simulink model "UZ_EnDat_be4_optimizing_agaib"  (R2023b)
settings: Solver=FixedStepDiscrete  StartTime=0  StopTime=0.002  RelTol=1e-3
model workspace (MAT data in the model file):
  Select = 0
libraries: hdlsllib x750, simulink x19, simulink_extras x4
(part 3 of 9)

== system UZ_EnDat_be4_optimizing_agaib/UZ_ENDAT/responseslicer5 ==
  DATA : Inport  OutDataTypeStr=uint64
  Bit Slice : hdlsllib/Logic and Bit Operations/Bit Slice  Commented=on  lidx=15  ridx=0
  Bit Slice1 : hdlsllib/Logic and Bit Operations/Bit Slice  Commented=on  lidx=63  ridx=48
  Bit Slice2 : hdlsllib/Logic and Bit Operations/Bit Slice  Commented=on  lidx=47  ridx=44
  Bit Slice3 : hdlsllib/Logic and Bit Operations/Bit Slice  lidx=43  ridx=39
  Bit Slice4 : hdlsllib/Logic and Bit Operations/Bit Slice  lidx=38  ridx=16
  Data Type Conversion : DataTypeConversion  Commented=on  OutDataTypeStr=uint16  SaturateOnIntegerOverflow=off  RndMeth=Floor
  Data Type Conversion1 : DataTypeConversion  Commented=on  OutDataTypeStr=uint16  SaturateOnIntegerOverflow=off  RndMeth=Floor
  Data Type Conversion2 : DataTypeConversion  Commented=through  OutDataTypeStr=uint8  SaturateOnIntegerOverflow=off  RndMeth=Floor
  Data Type Conversion3 : DataTypeConversion  OutDataTypeStr=uint8  SaturateOnIntegerOverflow=off  RndMeth=Floor
  Data Type Conversion4 : DataTypeConversion  OutDataTypeStr=uint32  SaturateOnIntegerOverflow=off  RndMeth=Floor
  ENDAT23BITREVERSER : Subsystem  Commented=on
  upppadding : Outport  OutDataTypeStr=uint16
  lowpadding : Outport  Port=2  OutDataTypeStr=uint16
  upperrecivervalue : Outport  Port=3  OutDataTypeStr=uint8
  CRC : Outport  Port=4  OutDataTypeStr=uint8
  payload : Outport  Port=5  OutDataTypeStr=uint32
  wires:
  DATA/1 -> Bit Slice4/1, Bit Slice3/1
  Bit Slice/1 -> Data Type Conversion/1
  Bit Slice1/1 -> Data Type Conversion1/1
  Data Type Conversion/1 -> lowpadding/1
  Data Type Conversion1/1 -> upppadding/1
  Bit Slice3/1 -> Data Type Conversion3/1
  Bit Slice2/1 -> Data Type Conversion2/1
  Bit Slice4/1 -> ENDAT23BITREVERSER/1(in), Data Type Conversion4/1
  Data Type Conversion2/1 -> upperrecivervalue/1
  Data Type Conversion3/1 -> CRC/1
  Data Type Conversion4/1 -> payload/1

== system UZ_EnDat_be4_optimizing_agaib/UZ_ENDAT/timingprovider ==
  wrok : Inport  OutDataTypeStr=boolean
  clk : Inport  Port=2  OutDataTypeStr=boolean
  CLKCNTER_POSCNTR : Subsystem
      settings: LibrarySourceBlock=|
      | hdlsllib/Ports &
      | Subsystems/Subsystem
  CLKCNTER_POSCNTR1 : Subsystem
      settings: LibrarySourceBlock=|
      | hdlsllib/Ports &
      | Subsystems/Subsystem
  Compare To Constant : hdlsllib/Logic and Bit Operations/Compare To Constant  relop=>  const=3  OutDataTypeStr=boolean
  Compare To Constant1 : hdlsllib/Logic and Bit Operations/Compare To Constant  relop===  const=0  OutDataTypeStr=boolean
  Constant3 : Constant  Commented=on  Value=0x7FFFF0  OutDataTypeStr=uint32  SampleTime=-1
  Constant4 : Constant  Commented=on  Value=0x7FFFFF  OutDataTypeStr=uint32  SampleTime=-1
  Detect Increase1 : simulink/Logic and Bit Operations/Detect Increase  vinit=0.0  OutDataTypeStr=boolean
      settings: LibrarySourceBlock=|
      | hdlsllib/Logic and Bit
      | Operations/Detect
      | Increase
  Logical Operator : Logic  Operator=OR  AllPortsSameDT=off  OutDataTypeStr=boolean
  Scope : Scope  NumInputPorts=2
  Subsystem2 : Subsystem
  Subsystem3 : Subsystem
  Subsystem4 : Subsystem  Commented=on
  timeelapsed2cycl : Outport  OutDataTypeStr=uint32
  timeelapsed1cycl : Outport  Port=2  OutDataTypeStr=uint32
  wires:
  clk/1 -> CLKCNTER_POSCNTR1/1(CLK), Subsystem4/1(countclk), CLKCNTER_POSCNTR/2(CLK2CNT), CLKCNTER_POSCNTR/1(CLK)
  wrok/1 -> Detect Increase1/1
  Detect Increase1/1 -> CLKCNTER_POSCNTR1/2(CLK2CNT)
  CLKCNTER_POSCNTR/1(CNT) -> Scope/1, Subsystem3/2(clkcnt), Subsystem2/2(clkcnt)
  Subsystem2/1(ns elapsed) -> timeelapsed2cycl/1
  Subsystem3/1(ns elapsed) -> Scope/2, timeelapsed1cycl/1
  CLKCNTER_POSCNTR1/1(CNT) -> Subsystem3/1(elapsed), Subsystem2/1(elapsed), Compare To Constant/1, Compare To Constant1/1
  Compare To Constant/1 -> Logical Operator/1, CLKCNTER_POSCNTR1/3(ResetCNT)
  Logical Operator/1 -> Subsystem4/2(reset), CLKCNTER_POSCNTR/3(ResetCNT)
  Compare To Constant1/1 -> Logical Operator/2

== system UZ_EnDat_be4_optimizing_agaib/UZ_ENDAT/3timestorage/Storage1 ==
  Data : Inport
  Write : Inport  Port=2  OutDataTypeStr=boolean
  Delay2 : Delay  DelayLength=1
  Switch : Switch  Criteria=u2 > Threshold  SaturateOnIntegerOverflow=off  InputSameDT=off
  out : Outport
  wires:
  Switch/1 -> Delay2/1, out/1
  Delay2/1 -> Switch/3
  Data/1 -> Switch/1
  Write/1 -> Switch/2

== system UZ_EnDat_be4_optimizing_agaib/UZ_ENDAT/3timestorage/Storage2 ==
  Data : Inport
  Write : Inport  Port=2  OutDataTypeStr=boolean
  Delay2 : Delay  DelayLength=1
  Switch : Switch  Criteria=u2 > Threshold  SaturateOnIntegerOverflow=off  InputSameDT=off
  out : Outport
  wires:
  Switch/1 -> Delay2/1, out/1
  Delay2/1 -> Switch/3
  Data/1 -> Switch/1
  Write/1 -> Switch/2

== system UZ_EnDat_be4_optimizing_agaib/UZ_ENDAT/3timestorage/Storage20 ==
  Data : Inport
  Write : Inport  Port=2  OutDataTypeStr=boolean
  Delay2 : Delay  DelayLength=1
  Switch : Switch  Criteria=u2 > Threshold  SaturateOnIntegerOverflow=off  InputSameDT=off
  out : Outport
  wires:
  Switch/1 -> Delay2/1, out/1
  Delay2/1 -> Switch/3
  Data/1 -> Switch/1
  Write/1 -> Switch/2

== system UZ_EnDat_be4_optimizing_agaib/UZ_ENDAT/3timestorage/Triggered Subsystem ==
  Trigger : TriggerPort  VariantControl=(inherit)
  Counter Limited : hdlsllib/Sources/Counter Limited  uplimit=2  tsamp=-1
  Out1 : Outport  InitialOutput=0
  wires:
  Counter Limited/1 -> Out1/1

== system UZ_EnDat_be4_optimizing_agaib/UZ_ENDAT/CLKCNTER_ACT/Positional_Counter ==
  valueout : Inport  OutDataTypeStr=uint32
  Trigger : TriggerPort  VariantControl=(inherit)  InitialTriggerSignalState=zero
  Increment Stored Integer : hdlsllib/Math Operations/Increment Stored Integer
  divider : Outport  InitialOutput=0
  wires:
  valueout/1 -> Increment Stored Integer/1
  Increment Stored Integer/1 -> divider/1

== system UZ_EnDat_be4_optimizing_agaib/UZ_ENDAT/CLKCNTER_ACT/SetZero32modified ==
  valin : Inport
  setzero : Inport  Port=2  OutDataTypeStr=boolean
  Trigger : TriggerPort  TriggerType=either  VariantControl=(inherit)
  Constant2 : Constant  Value=0  OutDataTypeStr=uint32  SampleTime=-1
  Index Vector1 : MultiPortSwitch  DataPortOrder=Zero-based contiguous  Inputs=2  zeroidx=on  SaturateOnIntegerOverflow=off  InputSameDT=off
  valueout : Outport  InitialOutput=1  VectorParamsAs1DForOutWhenUnconnected=off
  wires:
  valin/1 -> Index Vector1/2
  Index Vector1/1 -> valueout/1
  Constant2/1 -> Index Vector1/3
  setzero/1 -> Index Vector1/1

== system UZ_EnDat_be4_optimizing_agaib/UZ_ENDAT/CLKCNTER_NOSTOP/Positional_Counter ==
  valueout : Inport  OutDataTypeStr=uint32
  Trigger : TriggerPort  VariantControl=(inherit)  InitialTriggerSignalState=zero
  Increment Stored Integer : hdlsllib/Math Operations/Increment Stored Integer
  divider : Outport  InitialOutput=0
  wires:
  valueout/1 -> Increment Stored Integer/1
  Increment Stored Integer/1 -> divider/1

== system UZ_EnDat_be4_optimizing_agaib/UZ_ENDAT/CLKCNTER_NOSTOP/SetZero32modified ==
  valin : Inport
  setzero : Inport  Port=2  OutDataTypeStr=boolean
  Trigger : TriggerPort  TriggerType=either  VariantControl=(inherit)
  Constant2 : Constant  Value=0  OutDataTypeStr=uint32  SampleTime=-1
  Index Vector1 : MultiPortSwitch  DataPortOrder=Zero-based contiguous  Inputs=2  zeroidx=on  SaturateOnIntegerOverflow=off  InputSameDT=off
  valueout : Outport  InitialOutput=1  VectorParamsAs1DForOutWhenUnconnected=off
  wires:
  valin/1 -> Index Vector1/2
  Index Vector1/1 -> valueout/1
  Constant2/1 -> Index Vector1/3
  setzero/1 -> Index Vector1/1

== system UZ_EnDat_be4_optimizing_agaib/UZ_ENDAT/CLKDIV1/Triggered Subsystem ==
  IN : Inport
  Trigger : TriggerPort  VariantControl=(inherit)  OutputDataType=int8  InitialTriggerSignalState=positive
  OUT : Outport  InitialOutput=0
  wires:
  IN/1 -> OUT/1

== system UZ_EnDat_be4_optimizing_agaib/UZ_ENDAT/CLKDIV2/Triggered Subsystem ==
  IN : Inport
  Trigger : TriggerPort  VariantControl=(inherit)  OutputDataType=int8  InitialTriggerSignalState=positive
  OUT : Outport  InitialOutput=0
  wires:
  IN/1 -> OUT/1

== system UZ_EnDat_be4_optimizing_agaib/UZ_ENDAT/CLKDIV3/Triggered Subsystem ==
  IN : Inport
  Trigger : TriggerPort  VariantControl=(inherit)  OutputDataType=int8  InitialTriggerSignalState=positive
  OUT : Outport  InitialOutput=0
  wires:
  IN/1 -> OUT/1

== system UZ_EnDat_be4_optimizing_agaib/UZ_ENDAT/CLKDIV4/Triggered Subsystem ==
  IN : Inport
  Trigger : TriggerPort  VariantControl=(inherit)  OutputDataType=int8  InitialTriggerSignalState=positive
  OUT : Outport  InitialOutput=0
  wires:
  IN/1 -> OUT/1

== system UZ_EnDat_be4_optimizing_agaib/UZ_ENDAT/CLKDIV5/Triggered Subsystem ==
  IN : Inport
  Trigger : TriggerPort  VariantControl=(inherit)  OutputDataType=int8  InitialTriggerSignalState=positive
  OUT : Outport  InitialOutput=0
  wires:
  IN/1 -> OUT/1

== system UZ_EnDat_be4_optimizing_agaib/UZ_ENDAT/CLKDIV6/Triggered Subsystem ==
  IN : Inport
  Trigger : TriggerPort  VariantControl=(inherit)  OutputDataType=int8  InitialTriggerSignalState=positive
  OUT : Outport  InitialOutput=0
  wires:
  IN/1 -> OUT/1

== system UZ_EnDat_be4_optimizing_agaib/UZ_ENDAT/CLKDIV7/Triggered Subsystem ==
  IN : Inport
  Trigger : TriggerPort  VariantControl=(inherit)  OutputDataType=int8  InitialTriggerSignalState=positive
  OUT : Outport  InitialOutput=0
  wires:
  IN/1 -> OUT/1

== system UZ_EnDat_be4_optimizing_agaib/UZ_ENDAT/CLKDIV8/Triggered Subsystem ==
  IN : Inport
  Trigger : TriggerPort  VariantControl=(inherit)  OutputDataType=int8  InitialTriggerSignalState=positive
  OUT : Outport  InitialOutput=0
  wires:
  IN/1 -> OUT/1

== system UZ_EnDat_be4_optimizing_agaib/UZ_ENDAT/CLKDIV9/Triggered Subsystem ==
  IN : Inport
  Trigger : TriggerPort  VariantControl=(inherit)  OutputDataType=int8  InitialTriggerSignalState=positive
  OUT : Outport  InitialOutput=0
  wires:
  IN/1 -> OUT/1

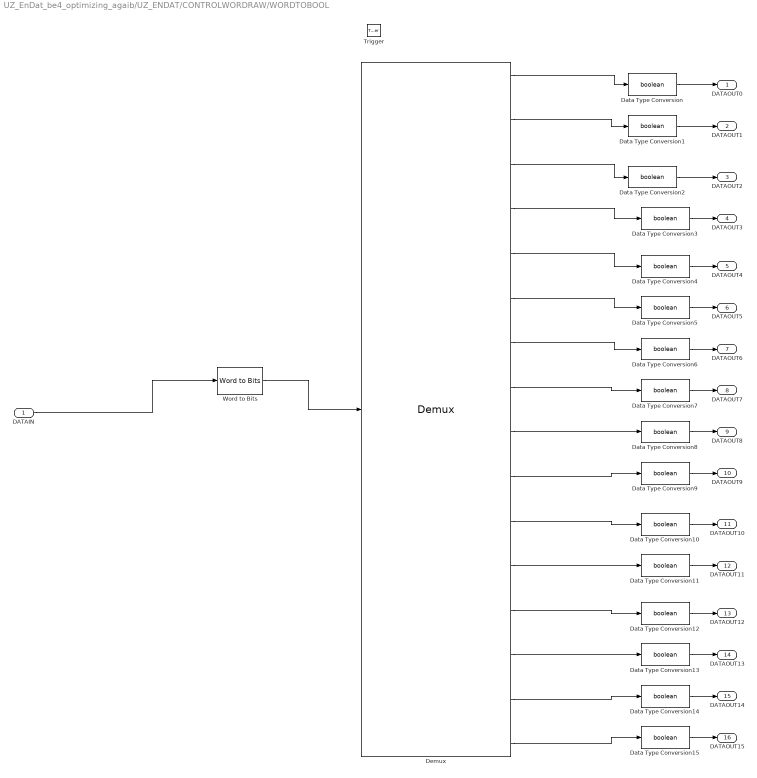
== system UZ_EnDat_be4_optimizing_agaib/UZ_ENDAT/CONTROLWORDRAW/WORDTOBOOL ==
  DATAIN : Inport
  Trigger : TriggerPort  TriggerType=falling  VariantControl=(inherit)  OutputDataType=int8  InitialTriggerSignalState=positive
  Data Type Conversion{,1..15} (16 alike) : DataTypeConversion  OutDataTypeStr=boolean  SaturateOnIntegerOverflow=off  RndMeth=Floor
  Demux : Demux  Outputs=16
  Word to Bits : hdlsllib/Logic and Bit Operations/Word to Bits  maxWordLength=16
  DATAOUT0 : Outport  InitialOutput=0
  DATAOUT1 : Outport  Port=2  InitialOutput=0
  DATAOUT2 : Outport  Port=3  InitialOutput=0
  DATAOUT3 : Outport  Port=4  InitialOutput=0
  DATAOUT4 : Outport  Port=5  InitialOutput=0
  DATAOUT5 : Outport  Port=6  InitialOutput=0
  DATAOUT6 : Outport  Port=7  InitialOutput=0
  DATAOUT7 : Outport  Port=8  InitialOutput=0
  DATAOUT8 : Outport  Port=9  InitialOutput=0
  DATAOUT9 : Outport  Port=10  InitialOutput=0
  DATAOUT10 : Outport  Port=11  InitialOutput=0
  DATAOUT11 : Outport  Port=12  InitialOutput=0
  DATAOUT12 : Outport  Port=13  InitialOutput=0
  DATAOUT13 : Outport  Port=14  InitialOutput=0
  DATAOUT14 : Outport  Port=15  InitialOutput=0
  DATAOUT15 : Outport  Port=16  InitialOutput=0
  wires:
  Demux/1 -> Data Type Conversion/1
  Demux/2 -> Data Type Conversion1/1
  Demux/4 -> Data Type Conversion3/1
  Demux/3 -> Data Type Conversion2/1
  Demux/6 -> Data Type Conversion5/1
  Demux/5 -> Data Type Conversion4/1
  Demux/8 -> Data Type Conversion7/1
  Demux/7 -> Data Type Conversion6/1
  Demux/10 -> Data Type Conversion9/1
  Demux/11 -> Data Type Conversion10/1
  Demux/12 -> Data Type Conversion11/1
  Demux/9 -> Data Type Conversion8/1
  Demux/13 -> Data Type Conversion12/1
  Demux/16 -> Data Type Conversion15/1
  Demux/14 -> Data Type Conversion13/1
  Demux/15 -> Data Type Conversion14/1
  Word to Bits/1 -> Demux/1
  Data Type Conversion/1 -> DATAOUT0/1
  Data Type Conversion1/1 -> DATAOUT1/1
  Data Type Conversion2/1 -> DATAOUT2/1
  Data Type Conversion3/1 -> DATAOUT3/1
  Data Type Conversion4/1 -> DATAOUT4/1
  Data Type Conversion5/1 -> DATAOUT5/1
  Data Type Conversion6/1 -> DATAOUT6/1
  Data Type Conversion7/1 -> DATAOUT7/1
  Data Type Conversion8/1 -> DATAOUT8/1
  Data Type Conversion9/1 -> DATAOUT9/1
  Data Type Conversion10/1 -> DATAOUT10/1
  Data Type Conversion11/1 -> DATAOUT11/1
  Data Type Conversion12/1 -> DATAOUT12/1
  Data Type Conversion13/1 -> DATAOUT13/1
  Data Type Conversion14/1 -> DATAOUT14/1
  Data Type Conversion15/1 -> DATAOUT15/1
  DATAIN/1 -> Word to Bits/1

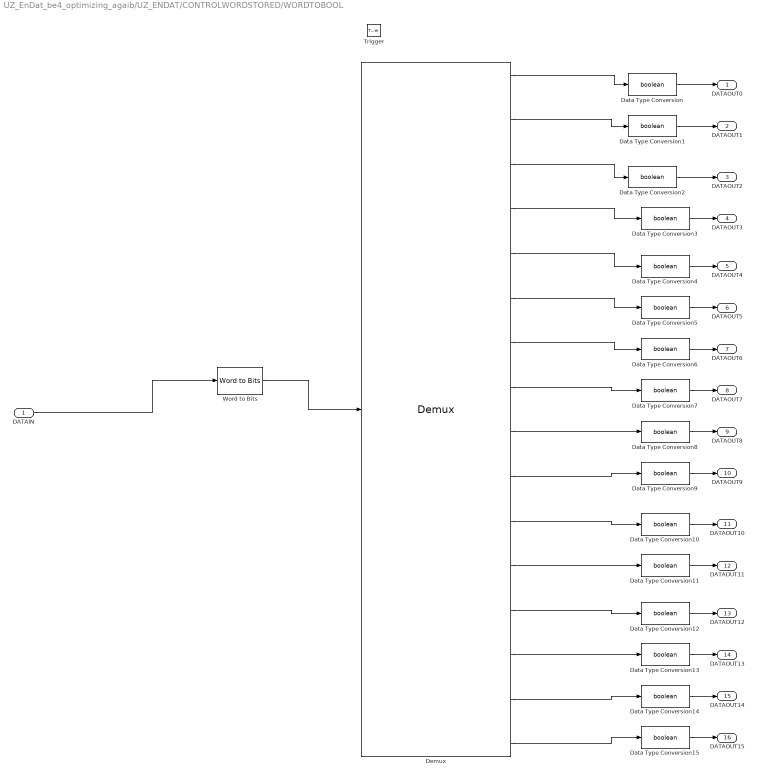
== system UZ_EnDat_be4_optimizing_agaib/UZ_ENDAT/CONTROLWORDSTORED/WORDTOBOOL ==
  DATAIN : Inport
  Trigger : TriggerPort  TriggerType=falling  VariantControl=(inherit)  OutputDataType=int8  InitialTriggerSignalState=positive
  Data Type Conversion{,1..15} (16 alike) : DataTypeConversion  OutDataTypeStr=boolean  SaturateOnIntegerOverflow=off  RndMeth=Floor
  Demux : Demux  Outputs=16
  Word to Bits : hdlsllib/Logic and Bit Operations/Word to Bits  maxWordLength=16
  DATAOUT0 : Outport  InitialOutput=0
  DATAOUT1 : Outport  Port=2  InitialOutput=0
  DATAOUT2 : Outport  Port=3  InitialOutput=0
  DATAOUT3 : Outport  Port=4  InitialOutput=0
  DATAOUT4 : Outport  Port=5  InitialOutput=0
  DATAOUT5 : Outport  Port=6  InitialOutput=0
  DATAOUT6 : Outport  Port=7  InitialOutput=0
  DATAOUT7 : Outport  Port=8  InitialOutput=0
  DATAOUT8 : Outport  Port=9  InitialOutput=0
  DATAOUT9 : Outport  Port=10  InitialOutput=0
  DATAOUT10 : Outport  Port=11  InitialOutput=0
  DATAOUT11 : Outport  Port=12  InitialOutput=0
  DATAOUT12 : Outport  Port=13  InitialOutput=0
  DATAOUT13 : Outport  Port=14  InitialOutput=0
  DATAOUT14 : Outport  Port=15  InitialOutput=0
  DATAOUT15 : Outport  Port=16  InitialOutput=0
  wires:
  Demux/1 -> Data Type Conversion/1
  Demux/2 -> Data Type Conversion1/1
  Demux/4 -> Data Type Conversion3/1
  Demux/3 -> Data Type Conversion2/1
  Demux/6 -> Data Type Conversion5/1
  Demux/5 -> Data Type Conversion4/1
  Demux/8 -> Data Type Conversion7/1
  Demux/7 -> Data Type Conversion6/1
  Demux/10 -> Data Type Conversion9/1
  Demux/11 -> Data Type Conversion10/1
  Demux/12 -> Data Type Conversion11/1
  Demux/9 -> Data Type Conversion8/1
  Demux/13 -> Data Type Conversion12/1
  Demux/16 -> Data Type Conversion15/1
  Demux/14 -> Data Type Conversion13/1
  Demux/15 -> Data Type Conversion14/1
  Word to Bits/1 -> Demux/1
  Data Type Conversion/1 -> DATAOUT0/1
  Data Type Conversion1/1 -> DATAOUT1/1
  Data Type Conversion2/1 -> DATAOUT2/1
  Data Type Conversion3/1 -> DATAOUT3/1
  Data Type Conversion4/1 -> DATAOUT4/1
  Data Type Conversion5/1 -> DATAOUT5/1
  Data Type Conversion6/1 -> DATAOUT6/1
  Data Type Conversion7/1 -> DATAOUT7/1
  Data Type Conversion8/1 -> DATAOUT8/1
  Data Type Conversion9/1 -> DATAOUT9/1
  Data Type Conversion10/1 -> DATAOUT10/1
  Data Type Conversion11/1 -> DATAOUT11/1
  Data Type Conversion12/1 -> DATAOUT12/1
  Data Type Conversion13/1 -> DATAOUT13/1
  Data Type Conversion14/1 -> DATAOUT14/1
  Data Type Conversion15/1 -> DATAOUT15/1
  DATAIN/1 -> Word to Bits/1

== system UZ_EnDat_be4_optimizing_agaib/UZ_ENDAT/CRC_Check/DFF1 ==
  SET : Inport
  CLK : Inport  Port=2
  D : Inport  Port=3
  RST : Inport  Port=4
  JKFF : Subsystem  TreatAsAtomicUnit=on
      settings: LibrarySourceBlock=|
      | hdlsllib/Ports &
      | Subsystems/Triggered
      | Subsystem
  NOT : Logic  Operator=NOT  IconShape=distinctive  AllPortsSameDT=off  OutDataTypeStr=boolean
  OQ : Outport
  NOQ : Outport  Port=2
  wires:
  SET/1 -> JKFF/1(SET)
  JKFF/2(NOQ) -> NOQ/1
  CLK/1 -> JKFF/2(CLK)
  JKFF/1(OQ) -> OQ/1
  RST/1 -> JKFF/4(RST)
  D/1 -> NOT/1, JKFF/3(J)
  NOT/1 -> JKFF/5(K)

== system UZ_EnDat_be4_optimizing_agaib/UZ_ENDAT/CRC_Check/DFF2 ==
  SET : Inport
  CLK : Inport  Port=2
  D : Inport  Port=3
  RST : Inport  Port=4
  JKFF : Subsystem  TreatAsAtomicUnit=on
      settings: LibrarySourceBlock=|
      | hdlsllib/Ports &
      | Subsystems/Triggered
      | Subsystem
  NOT : Logic  Operator=NOT  IconShape=distinctive  AllPortsSameDT=off  OutDataTypeStr=boolean
  OQ : Outport
  NOQ : Outport  Port=2
  wires:
  SET/1 -> JKFF/1(SET)
  JKFF/2(NOQ) -> NOQ/1
  CLK/1 -> JKFF/2(CLK)
  JKFF/1(OQ) -> OQ/1
  RST/1 -> JKFF/4(RST)
  D/1 -> NOT/1, JKFF/3(J)
  NOT/1 -> JKFF/5(K)

== system UZ_EnDat_be4_optimizing_agaib/UZ_ENDAT/CRC_Check/DFF3 ==
  SET : Inport
  CLK : Inport  Port=2
  D : Inport  Port=3
  RST : Inport  Port=4
  JKFF : Subsystem  TreatAsAtomicUnit=on
      settings: LibrarySourceBlock=|
      | hdlsllib/Ports &
      | Subsystems/Triggered
      | Subsystem
  NOT : Logic  Operator=NOT  IconShape=distinctive  AllPortsSameDT=off  OutDataTypeStr=boolean
  OQ : Outport
  NOQ : Outport  Port=2
  wires:
  SET/1 -> JKFF/1(SET)
  JKFF/2(NOQ) -> NOQ/1
  CLK/1 -> JKFF/2(CLK)
  JKFF/1(OQ) -> OQ/1
  RST/1 -> JKFF/4(RST)
  D/1 -> NOT/1, JKFF/3(J)
  NOT/1 -> JKFF/5(K)

== system UZ_EnDat_be4_optimizing_agaib/UZ_ENDAT/CRC_Check/DFF4 ==
  SET : Inport
  CLK : Inport  Port=2
  D : Inport  Port=3
  RST : Inport  Port=4
  JKFF : Subsystem  TreatAsAtomicUnit=on
      settings: LibrarySourceBlock=|
      | hdlsllib/Ports &
      | Subsystems/Triggered
      | Subsystem
  NOT : Logic  Operator=NOT  IconShape=distinctive  AllPortsSameDT=off  OutDataTypeStr=boolean
  OQ : Outport
  NOQ : Outport  Port=2
  wires:
  SET/1 -> JKFF/1(SET)
  JKFF/2(NOQ) -> NOQ/1
  CLK/1 -> JKFF/2(CLK)
  JKFF/1(OQ) -> OQ/1
  RST/1 -> JKFF/4(RST)
  D/1 -> NOT/1, JKFF/3(J)
  NOT/1 -> JKFF/5(K)

== system UZ_EnDat_be4_optimizing_agaib/UZ_ENDAT/CRC_Check/DFF5 ==
  SET : Inport
  CLK : Inport  Port=2
  D : Inport  Port=3
  RST : Inport  Port=4
  JKFF : Subsystem  TreatAsAtomicUnit=on
      settings: LibrarySourceBlock=|
      | hdlsllib/Ports &
      | Subsystems/Triggered
      | Subsystem
  NOT : Logic  Operator=NOT  IconShape=distinctive  AllPortsSameDT=off  OutDataTypeStr=boolean
  OQ : Outport
  NOQ : Outport  Port=2
  wires:
  SET/1 -> JKFF/1(SET)
  JKFF/2(NOQ) -> NOQ/1
  CLK/1 -> JKFF/2(CLK)
  JKFF/1(OQ) -> OQ/1
  RST/1 -> JKFF/4(RST)
  D/1 -> NOT/1, JKFF/3(J)
  NOT/1 -> JKFF/5(K)

== system UZ_EnDat_be4_optimizing_agaib/UZ_ENDAT/CRC_Check/DFF6 ==
  SET : Inport
  CLK : Inport  Port=2
  D : Inport  Port=3
  RST : Inport  Port=4
  JKFF : Subsystem  TreatAsAtomicUnit=on
      settings: LibrarySourceBlock=|
      | hdlsllib/Ports &
      | Subsystems/Triggered
      | Subsystem
  NOT : Logic  Operator=NOT  IconShape=distinctive  AllPortsSameDT=off  OutDataTypeStr=boolean
  OQ : Outport
  NOQ : Outport  Port=2
  wires:
  SET/1 -> JKFF/1(SET)
  JKFF/2(NOQ) -> NOQ/1
  CLK/1 -> JKFF/2(CLK)
  JKFF/1(OQ) -> OQ/1
  RST/1 -> JKFF/4(RST)
  D/1 -> NOT/1, JKFF/3(J)
  NOT/1 -> JKFF/5(K)

== system UZ_EnDat_be4_optimizing_agaib/UZ_ENDAT/CRC_Check/FF0 ==
  SET : Inport
  CLK : Inport  Port=2
  DATA : Inport  Port=3
  RST : Inport  Port=4
  Delay{,1..5} (6 alike) : Delay  DelayLength=1
  Logical Operator{,1..5} (6 alike) : Logic  Operator=NAND  Inputs=3  AllPortsSameDT=off  OutDataTypeStr=boolean
  OQ : Outport
  NOQ : Outport  Port=2
  wires:
  SET/1 -> Logical Operator/1, Logical Operator4/1
  Logical Operator/1 -> Delay/1
  Logical Operator1/1 -> Delay1/1
  DATA/1 -> Logical Operator3/2
  RST/1 -> Logical Operator1/3, Logical Operator5/3, Logical Operator3/3
  Logical Operator4/1 -> Delay4/1
  Logical Operator5/1 -> Delay5/1
  Logical Operator2/1 -> Delay2/1
  Logical Operator3/1 -> Delay3/1
  CLK/1 -> Logical Operator2/2, Logical Operator1/2
  Delay/1 -> Logical Operator1/1
  Delay1/1 -> Logical Operator4/2, Logical Operator2/1, Logical Operator/3
  Delay2/1 -> Logical Operator3/1, Logical Operator5/2
  Delay3/1 -> Logical Operator/2, Logical Operator2/3
  Delay4/1 -> Logical Operator5/1, OQ/1
  Delay5/1 -> NOQ/1, Logical Operator4/3

== system UZ_EnDat_be4_optimizing_agaib/UZ_ENDAT/INITIALOFF/CLKCNTER_FAST ==
  CLK : Inport
  Delay1 : Delay  DelayLength=1
  Positional_Counter : Subsystem  TreatAsAtomicUnit=on
      settings: LibrarySourceBlock=|
      | hdlsllib/Ports &
      | Subsystems/Triggered
      | Subsystem
  CNT : Outport
  wires:
  Delay1/1 -> Positional_Counter/1(valueout), CNT/1
  CLK/1 -> Positional_Counter/Trigger
  Positional_Counter/1(divider) -> Delay1/1

== system UZ_EnDat_be4_optimizing_agaib/UZ_ENDAT/INITIALOFF/Subsystem6 ==
  FACTOR : Inport  OutMin=0  OutMax=60000
  Add1 : Sum  Inputs=+-  OutDataTypeStr=uint16  AccumDataTypeStr=uint16  RndMeth=Simplest  SaturateOnIntegerOverflow=on
  Add2 : Sum  OutDataTypeStr=uint16  AccumDataTypeStr=int16  RndMeth=Simplest  SaturateOnIntegerOverflow=on
  Add3 : Sum  Inputs=+-  OutDataTypeStr=uint16  AccumDataTypeStr=uint16  RndMeth=Simplest  SaturateOnIntegerOverflow=on
  Compare To Constant : hdlsllib/Logic and Bit Operations/Compare To Constant  relop=<  const=100  OutDataTypeStr=boolean
  Constant : Constant  Value=20  OutDataTypeStr=int16  SampleTime=-1
  Constant1 : Constant  Value=-20  OutDataTypeStr=int16  SampleTime=-1
  Constant2 : Constant  Value=100  OutDataTypeStr=uint16  SampleTime=-1
  Constant3 : Constant  Value=2000  OutDataTypeStr=uint16  SampleTime=-1
  Display : Display
  Display1 : Display
  Product : Product  OutDataTypeStr=int32
  Switch : Switch  Criteria=u2 > Threshold  SaturateOnIntegerOverflow=off  InputSameDT=off
  Switch1 : Switch  Criteria=u2 > Threshold  SaturateOnIntegerOverflow=off  InputSameDT=off
  out : Outport
  wires:
  FACTOR/1 -> Add3/1, Add1/2, Compare To Constant/1
  Constant2/1 -> Add1/1, Add3/2
  Compare To Constant/1 -> Switch1/2, Switch/2
  Constant1/1 -> Switch1/1
  Add1/1 -> Switch/1
  Switch/1 -> Product/1
  Constant/1 -> Switch1/3
  Switch1/1 -> Product/2
  Constant3/1 -> Add2/1
  Product/1 -> Add2/2, Display1/1
  Add2/1 -> Display/1, out/1
  Add3/1 -> Switch/3

== system UZ_EnDat_be4_optimizing_agaib/UZ_ENDAT/ManualSerialize/FF1 ==
  SET : Inport
  RST : Inport  Port=2
  S-R Flip-Flop : simulink_extras/Flip Flops/S-R Flip-Flop  initial_condition=0
  OQ : Outport
  NOQ : Outport  Port=2
  wires:
  SET/1 -> S-R Flip-Flop/1
  RST/1 -> S-R Flip-Flop/2
  S-R Flip-Flop/1 -> OQ/1
  S-R Flip-Flop/2 -> NOQ/1

== system UZ_EnDat_be4_optimizing_agaib/UZ_ENDAT/ManualSerialize/SetZero64modified ==
  valin : Inport
  setzero : Inport  Port=2  OutDataTypeStr=boolean
  Trigger : TriggerPort  TriggerType=either  VariantControl=(inherit)
  Constant2 : Constant  Value=0  OutDataTypeStr=uint64  SampleTime=-1
  Index Vector1 : MultiPortSwitch  DataPortOrder=Zero-based contiguous  Inputs=2  zeroidx=on  OutDataTypeStr=uint64  SaturateOnIntegerOverflow=off  InputSameDT=off
  valueout : Outport  InitialOutput=1  VectorParamsAs1DForOutWhenUnconnected=off
  wires:
  valin/1 -> Index Vector1/2
  Index Vector1/1 -> valueout/1
  Constant2/1 -> Index Vector1/3
  setzero/1 -> Index Vector1/1

== system UZ_EnDat_be4_optimizing_agaib/UZ_ENDAT/ManualSerialize/Storage1 ==
  Data : Inport
  Write : Inport  Port=2  OutDataTypeStr=boolean
  Compare To Zero : hdlsllib/Logic and Bit Operations/Compare To Zero  relop=>  OutDataTypeStr=boolean
  Logical Operator1 : Logic  AllPortsSameDT=off  OutDataTypeStr=boolean
  out : Outport
  wrok : Outport  Port=2  OutDataTypeStr=boolean
  wires:
  Compare To Zero/1 -> Logical Operator1/2
  Logical Operator1/1 -> wrok/1
  Data/1 -> out/1, Compare To Zero/1
  Write/1 -> Logical Operator1/1

== system UZ_EnDat_be4_optimizing_agaib/UZ_ENDAT/ManualSerialize/Storage16 ==
  Data : Inport
  Write : Inport  Port=2  OutDataTypeStr=boolean
  Compare To Zero : hdlsllib/Logic and Bit Operations/Compare To Zero  relop===  OutDataTypeStr=boolean
  Logical Operator : Logic  Operator=NOT  AllPortsSameDT=off  OutDataTypeStr=boolean
  Logical Operator1 : Logic  Inputs=3  AllPortsSameDT=off  OutDataTypeStr=boolean
  Logical Operator2 : Logic  Operator=NOT  AllPortsSameDT=off  OutDataTypeStr=boolean
  Logical Operator3 : Logic  Inputs=3  AllPortsSameDT=off  OutDataTypeStr=boolean
  Logical Operator4 : Logic  Operator=NOT  AllPortsSameDT=off  OutDataTypeStr=boolean
  Relational Operator : RelationalOperator  Operator===  OutDataTypeStr=boolean  InputSameDT=off
  Scope : Scope  NumInputPorts=5
  Single Port RAM System : hdlsllib/HDL RAMs/Single Port RAM System  RAMType=Single port  AsyncRead=off  WriteOutputValue=Old data  RAMInitialValue=0  allowBusInputs=off  WritesHaveOutput=on  NumReads=0  NumWrites=1  SimulateUsing=Code generation
  adress : Constant  Value=6  OutDataTypeStr=uint8  SampleTime=-1
  out : Outport
  wrok : Outport  Port=2  OutDataTypeStr=boolean
  wires:
  Single Port RAM System/1 -> Relational Operator/1, out/1
  Data/1 -> Compare To Zero/1, Single Port RAM System/1, Relational Operator/2
  adress/1 -> Single Port RAM System/2
  Relational Operator/1 -> Scope/1, Logical Operator/1, Logical Operator3/1
  Logical Operator/1 -> Logical Operator1/2
  Write/1 -> Scope/4, Logical Operator4/1, Logical Operator1/1
  Compare To Zero/1 -> Logical Operator2/1
  Logical Operator1/1 -> Single Port RAM System/3, Scope/5
  Logical Operator3/1 -> wrok/1, Scope/2
  Logical Operator4/1 -> Logical Operator3/3
  Logical Operator2/1 -> Logical Operator1/3, Logical Operator3/2, Scope/3

== system UZ_EnDat_be4_optimizing_agaib/UZ_ENDAT/ManualSerialize/Storage2 ==
  Data : Inport
  Write : Inport  Port=2  OutDataTypeStr=boolean
  Compare To Zero : hdlsllib/Logic and Bit Operations/Compare To Zero  relop===  OutDataTypeStr=boolean
  Delay : Delay  DelayLength=1
  Delay2 : Delay  DelayLength=1
  Logical Operator1 : Logic  AllPortsSameDT=off  OutDataTypeStr=boolean
  Logical Operator2 : Logic  Operator=NOT  AllPortsSameDT=off  OutDataTypeStr=boolean
  Scope1 : Scope  NumInputPorts=2
  Single Port RAM System : hdlsllib/HDL RAMs/Single Port RAM System  Commented=on  RAMType=Single port  AsyncRead=off  WriteOutputValue=Old data  RAMInitialValue=0  allowBusInputs=off  WritesHaveOutput=on  NumReads=0  NumWrites=1  SimulateUsing=Code generation
  Switch : Switch  Criteria=u2 > Threshold  SaturateOnIntegerOverflow=off  InputSameDT=off
  prolonger : Subsystem
  out : Outport
  wrok : Outport  Port=2  OutDataTypeStr=boolean
  wires:
  Switch/1 -> Delay2/1
  Compare To Zero/1 -> Logical Operator2/1
  Logical Operator1/1 -> Delay/1, Switch/2
  Logical Operator2/1 -> Logical Operator1/2
  prolonger/1(out) -> wrok/1
  Data/1 -> Scope1/1, Compare To Zero/1, Switch/1
  Delay2/1 -> out/1, Switch/3
  Delay/1 -> prolonger/1(in)
  Write/1 -> Logical Operator1/1

== system UZ_EnDat_be4_optimizing_agaib/UZ_ENDAT/ManualSerialize/Subsystem ==
  countclk : Inport
  reset : Inport  Port=2
  Delay : Delay  DelayLength=1
  Detect Increase : simulink/Logic and Bit Operations/Detect Increase  vinit=0.0  OutDataTypeStr=boolean
      settings: LibrarySourceBlock=|
      | hdlsllib/Logic and Bit
      | Operations/Detect
      | Increase
  HDL Counter : hdlsllib/Sources/HDL Counter  CountType=Count limited  CountInit=0  CountStep=1  CountMax=51  CountFromType=Initial value  CountFrom=0  CountResetPort=on  CountLoadPort=off  CountEnbPort=on  CountDirPort=off  CountHitOutputPort=off  CountDataType=Unsigned  CountWordLen=8  CountFracLen=0  CountSampTime=1
  valin1 : Outport  InitialOutput=0
  wires:
  countclk/1 -> Detect Increase/1
  Detect Increase/1 -> HDL Counter/2
  reset/1 -> Delay/1
  HDL Counter/1 -> valin1/1
  Delay/1 -> HDL Counter/1

== system UZ_EnDat_be4_optimizing_agaib/UZ_ENDAT/ManualSerialize/Triggered Subsystem ==
  DATA : Inport
  valueout : Inport  Port=2
  Trigger : TriggerPort  VariantControl=(inherit)
  Bit Clear : simulink/Logic and Bit Operations/Bit Clear  iBit=50
      settings: LibrarySourceBlock=|
      | hdlsllib/Logic and Bit
      | Operations/Bit Clear
  Bit Set : simulink/Logic and Bit Operations/Bit Set  iBit=50
      settings: LibrarySourceBlock=|
      | hdlsllib/Logic and Bit
      | Operations/Bit Set
  Bit Shift : hdlsllib/Logic and Bit Operations/Bit Shift  mode=Shift Right Logical  N=1
  Display : Display
      settings: Format=binary (Stored Integer)
  Scope : Scope  NumInputPorts=2
  Switch : Switch  Criteria=u2 ~= 0  SaturateOnIntegerOverflow=off  InputSameDT=off
  valin : Outport  InitialOutput=0
  wires:
  DATA/1 -> Scope/1, Switch/2
  valueout/1 -> Bit Clear/1, Bit Set/1, Scope/2
  Bit Set/1 -> Switch/1
  Switch/1 -> Bit Shift/1
  Bit Shift/1 -> Display/1, valin/1
  Bit Clear/1 -> Switch/3

== system UZ_EnDat_be4_optimizing_agaib/UZ_ENDAT/ManualSerialize/nibblepadding6 ==
  in : Inport
  padding : Subsystem
  padding1 : Subsystem
  padding2 : Subsystem
  padding3 : Subsystem
  out : Outport
  wires:
  in/1 -> padding3/1(in)
  padding2/1(out) -> padding1/1(in)
  padding3/1(out) -> padding2/1(in)
  padding1/1(out) -> padding/1(in)
  padding/1(out) -> out/1

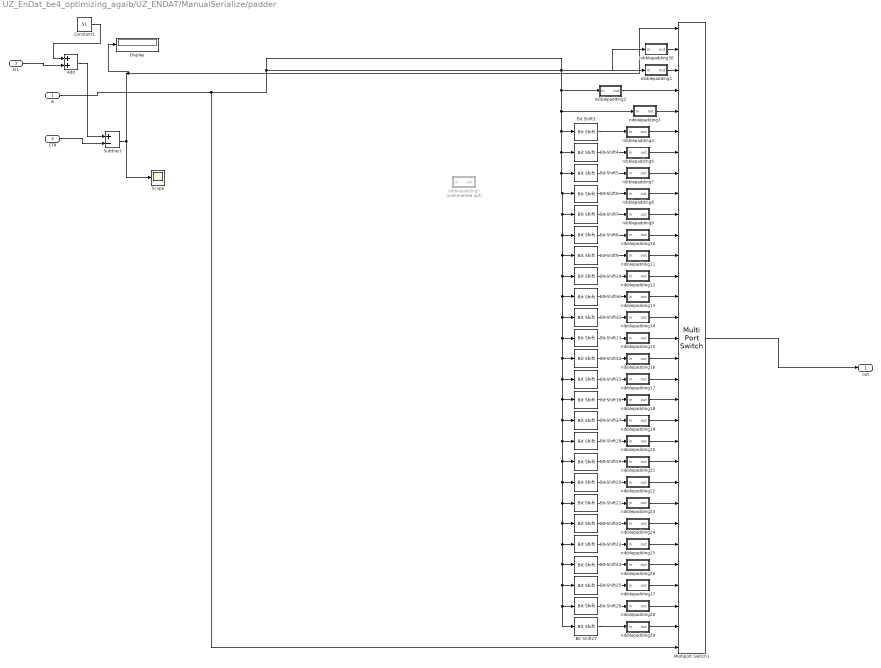
== system UZ_EnDat_be4_optimizing_agaib/UZ_ENDAT/ManualSerialize/padder ==
  in : Inport
  CTR : Inport  Port=2
  in1 : Inport  Port=3  OutDataTypeStr=int8
  Add : Sum  OutDataTypeStr=uint8  AccumDataTypeStr=uint8  RndMeth=Simplest
  Bit Shift10 : hdlsllib/Logic and Bit Operations/Bit Shift  mode=Shift Right Logical  N=8
  Bit Shift11 : hdlsllib/Logic and Bit Operations/Bit Shift  mode=Shift Right Logical  N=9
  Bit Shift12 : hdlsllib/Logic and Bit Operations/Bit Shift  mode=Shift Right Logical  N=10
  Bit Shift13 : hdlsllib/Logic and Bit Operations/Bit Shift  mode=Shift Right Logical  N=11
  Bit Shift14 : hdlsllib/Logic and Bit Operations/Bit Shift  mode=Shift Right Logical  N=12
  Bit Shift15 : hdlsllib/Logic and Bit Operations/Bit Shift  mode=Shift Right Logical  N=13
  Bit Shift16 : hdlsllib/Logic and Bit Operations/Bit Shift  mode=Shift Right Logical  N=14
  Bit Shift17 : hdlsllib/Logic and Bit Operations/Bit Shift  mode=Shift Right Logical  N=15
  Bit Shift18 : hdlsllib/Logic and Bit Operations/Bit Shift  mode=Shift Right Logical  N=16
  Bit Shift19 : hdlsllib/Logic and Bit Operations/Bit Shift  mode=Shift Right Logical  N=17
  Bit Shift20 : hdlsllib/Logic and Bit Operations/Bit Shift  mode=Shift Right Logical  N=18
  Bit Shift21 : hdlsllib/Logic and Bit Operations/Bit Shift  mode=Shift Right Logical  N=19
  Bit Shift22 : hdlsllib/Logic and Bit Operations/Bit Shift  mode=Shift Right Logical  N=20
  Bit Shift23 : hdlsllib/Logic and Bit Operations/Bit Shift  mode=Shift Right Logical  N=21
  Bit Shift24 : hdlsllib/Logic and Bit Operations/Bit Shift  mode=Shift Right Logical  N=22
  Bit Shift25 : hdlsllib/Logic and Bit Operations/Bit Shift  mode=Shift Right Logical  N=23
  Bit Shift26 : hdlsllib/Logic and Bit Operations/Bit Shift  mode=Shift Right Logical  N=24
  Bit Shift27 : hdlsllib/Logic and Bit Operations/Bit Shift  mode=Shift Right Logical  N=25
  Bit Shift3 : hdlsllib/Logic and Bit Operations/Bit Shift  mode=Shift Right Logical  N=1
  Bit Shift4 : hdlsllib/Logic and Bit Operations/Bit Shift  mode=Shift Right Logical  N=2
  Bit Shift5 : hdlsllib/Logic and Bit Operations/Bit Shift  mode=Shift Right Logical  N=3
  Bit Shift6 : hdlsllib/Logic and Bit Operations/Bit Shift  mode=Shift Right Logical  N=4
  Bit Shift7 : hdlsllib/Logic and Bit Operations/Bit Shift  mode=Shift Right Logical  N=5
  Bit Shift8 : hdlsllib/Logic and Bit Operations/Bit Shift  mode=Shift Right Logical  N=6
  Bit Shift9 : hdlsllib/Logic and Bit Operations/Bit Shift  mode=Shift Right Logical  N=7
  Constant1 : Constant  Value=51  OutDataTypeStr=uint8  SampleTime=-1
  Display : Display
  Multiport Switch1 : MultiPortSwitch  DataPortOrder=Zero-based contiguous  Inputs=29  DataPortForDefault=Additional data port  DiagnosticForDefault=Warning  zeroidx=on  RndMeth=Simplest  SaturateOnIntegerOverflow=off  InputSameDT=off
  Scope : Scope
  Subtract : Sum  Inputs=+-  OutDataTypeStr=uint8  AccumDataTypeStr=uint8  RndMeth=Simplest  SaturateOnIntegerOverflow=on
  nibblepadding1 : Subsystem
  nibblepadding10 : Subsystem
  nibblepadding11 : Subsystem
  nibblepadding12 : Subsystem
  nibblepadding13 : Subsystem
  nibblepadding14 : Subsystem
  nibblepadding15 : Subsystem
  nibblepadding16 : Subsystem
  nibblepadding17 : Subsystem
  nibblepadding18 : Subsystem
  nibblepadding19 : Subsystem
  nibblepadding2 : Subsystem
  nibblepadding20 : Subsystem
  nibblepadding21 : Subsystem
  nibblepadding22 : Subsystem
  nibblepadding23 : Subsystem
  nibblepadding24 : Subsystem
  nibblepadding25 : Subsystem
  nibblepadding26 : Subsystem
  nibblepadding27 : Subsystem
  nibblepadding28 : Subsystem
  nibblepadding29 : Subsystem
  nibblepadding3 : Subsystem
  nibblepadding30 : Subsystem
  nibblepadding4 : Subsystem
  nibblepadding5 : Subsystem  Commented=on
  nibblepadding6 : Subsystem
  nibblepadding7 : Subsystem
  nibblepadding8 : Subsystem
  nibblepadding9 : Subsystem
  out : Outport
  wires:
  Multiport Switch1/1 -> out/1
  CTR/1 -> Subtract/2
  Bit Shift27/1 -> nibblepadding29/1(in)
  Bit Shift26/1 -> nibblepadding28/1(in)
  Bit Shift25/1 -> nibblepadding27/1(in)
  Bit Shift24/1 -> nibblepadding26/1(in)
  Bit Shift23/1 -> nibblepadding25/1(in)
  Bit Shift22/1 -> nibblepadding24/1(in)
  Bit Shift21/1 -> nibblepadding23/1(in)
  Bit Shift20/1 -> nibblepadding22/1(in)
  Bit Shift19/1 -> nibblepadding21/1(in)
  Bit Shift18/1 -> nibblepadding20/1(in)
  Bit Shift17/1 -> nibblepadding19/1(in)
  Bit Shift16/1 -> nibblepadding18/1(in)
  Bit Shift15/1 -> nibblepadding17/1(in)
  Bit Shift14/1 -> nibblepadding16/1(in)
  Bit Shift13/1 -> nibblepadding15/1(in)
  Bit Shift12/1 -> nibblepadding14/1(in)
  Bit Shift11/1 -> nibblepadding13/1(in)
  Bit Shift10/1 -> nibblepadding12/1(in)
  Bit Shift9/1 -> nibblepadding11/1(in)
  Bit Shift8/1 -> nibblepadding10/1(in)
  Bit Shift7/1 -> nibblepadding9/1(in)
  Bit Shift6/1 -> nibblepadding8/1(in)
  Bit Shift5/1 -> nibblepadding7/1(in)
  Bit Shift4/1 -> nibblepadding6/1(in)
  Bit Shift3/1 -> nibblepadding4/1(in)
  in/1 -> Multiport Switch1/31, nibblepadding1/1(in), nibblepadding2/1(in), nibblepadding3/1(in), Bit Shift26/1, Bit Shift27/1, Bit Shift25/1, Bit Shift24/1, Bit Shift23/1, Bit Shift22/1, Bit Shift21/1, Bit Shift20/1, Bit Shift19/1, Bit Shift18/1, Bit Shift17/1, Bit Shift16/1, Bit Shift15/1, Bit Shift14/1, Bit Shift13/1, Bit Shift12/1, Bit Shift11/1, Bit Shift10/1, Bit Shift9/1, Bit Shift8/1, Bit Shift7/1, Bit Shift6/1, Bit Shift5/1, Bit Shift4/1, Bit Shift3/1, nibblepadding30/1(in)
  in1/1 -> Add/2
  Constant1/1 -> Add/1
  Subtract/1 -> Display/1, Multiport Switch1/1, Scope/1
  Add/1 -> Subtract/1
  nibblepadding1/1(out) -> Multiport Switch1/3
  nibblepadding2/1(out) -> Multiport Switch1/4
  nibblepadding3/1(out) -> Multiport Switch1/5
  nibblepadding4/1(out) -> Multiport Switch1/6
  nibblepadding6/1(out) -> Multiport Switch1/7
  nibblepadding7/1(out) -> Multiport Switch1/8
  nibblepadding8/1(out) -> Multiport Switch1/9
  nibblepadding9/1(out) -> Multiport Switch1/10
  nibblepadding10/1(out) -> Multiport Switch1/11
  nibblepadding11/1(out) -> Multiport Switch1/12
  nibblepadding29/1(out) -> Multiport Switch1/30
  nibblepadding28/1(out) -> Multiport Switch1/29
  nibblepadding27/1(out) -> Multiport Switch1/28
  nibblepadding26/1(out) -> Multiport Switch1/27
  nibblepadding25/1(out) -> Multiport Switch1/26
  nibblepadding24/1(out) -> Multiport Switch1/25
  nibblepadding23/1(out) -> Multiport Switch1/24
  nibblepadding22/1(out) -> Multiport Switch1/23
  nibblepadding21/1(out) -> Multiport Switch1/22
  nibblepadding20/1(out) -> Multiport Switch1/21
  nibblepadding19/1(out) -> Multiport Switch1/20
  nibblepadding18/1(out) -> Multiport Switch1/19
  nibblepadding17/1(out) -> Multiport Switch1/18
  nibblepadding16/1(out) -> Multiport Switch1/17
  nibblepadding15/1(out) -> Multiport Switch1/16
  nibblepadding14/1(out) -> Multiport Switch1/15
  nibblepadding13/1(out) -> Multiport Switch1/14
  nibblepadding12/1(out) -> Multiport Switch1/13
  nibblepadding30/1(out) -> Multiport Switch1/2

== system UZ_EnDat_be4_optimizing_agaib/UZ_ENDAT/ManualSerialize/padder1 ==
  in : Inport
  CTR : Inport  Port=2
  in1 : Inport  Port=3  OutDataTypeStr=int8
  Add : Sum  OutDataTypeStr=uint8  AccumDataTypeStr=uint8  RndMeth=Simplest
  Bit Shift10 : hdlsllib/Logic and Bit Operations/Bit Shift  mode=Shift Right Logical  N=8
  Bit Shift11 : hdlsllib/Logic and Bit Operations/Bit Shift  mode=Shift Right Logical  N=9
  Bit Shift12 : hdlsllib/Logic and Bit Operations/Bit Shift  mode=Shift Right Logical  N=10
  Bit Shift13 : hdlsllib/Logic and Bit Operations/Bit Shift  mode=Shift Right Logical  N=11
  Bit Shift14 : hdlsllib/Logic and Bit Operations/Bit Shift  mode=Shift Right Logical  N=12
  Bit Shift15 : hdlsllib/Logic and Bit Operations/Bit Shift  mode=Shift Right Logical  N=13
  Bit Shift16 : hdlsllib/Logic and Bit Operations/Bit Shift  mode=Shift Right Logical  N=14
  Bit Shift17 : hdlsllib/Logic and Bit Operations/Bit Shift  mode=Shift Right Logical  N=15
  Bit Shift18 : hdlsllib/Logic and Bit Operations/Bit Shift  mode=Shift Right Logical  N=16
  Bit Shift19 : hdlsllib/Logic and Bit Operations/Bit Shift  mode=Shift Right Logical  N=17
  Bit Shift20 : hdlsllib/Logic and Bit Operations/Bit Shift  mode=Shift Right Logical  N=18
  Bit Shift21 : hdlsllib/Logic and Bit Operations/Bit Shift  mode=Shift Right Logical  N=19
  Bit Shift22 : hdlsllib/Logic and Bit Operations/Bit Shift  mode=Shift Right Logical  N=20
  Bit Shift23 : hdlsllib/Logic and Bit Operations/Bit Shift  mode=Shift Right Logical  N=21
  Bit Shift24 : hdlsllib/Logic and Bit Operations/Bit Shift  mode=Shift Right Logical  N=22
  Bit Shift25 : hdlsllib/Logic and Bit Operations/Bit Shift  mode=Shift Right Logical  N=23
  Bit Shift26 : hdlsllib/Logic and Bit Operations/Bit Shift  mode=Shift Right Logical  N=24
  Bit Shift27 : hdlsllib/Logic and Bit Operations/Bit Shift  mode=Shift Right Logical  N=25
  Bit Shift3 : hdlsllib/Logic and Bit Operations/Bit Shift  mode=Shift Right Logical  N=1
  Bit Shift4 : hdlsllib/Logic and Bit Operations/Bit Shift  mode=Shift Right Logical  N=2
  Bit Shift5 : hdlsllib/Logic and Bit Operations/Bit Shift  mode=Shift Right Logical  N=3
  Bit Shift6 : hdlsllib/Logic and Bit Operations/Bit Shift  mode=Shift Right Logical  N=4
  Bit Shift7 : hdlsllib/Logic and Bit Operations/Bit Shift  mode=Shift Right Logical  N=5
  Bit Shift8 : hdlsllib/Logic and Bit Operations/Bit Shift  mode=Shift Right Logical  N=6
  Bit Shift9 : hdlsllib/Logic and Bit Operations/Bit Shift  mode=Shift Right Logical  N=7
  Constant1 : Constant  Value=51  OutDataTypeStr=uint8  SampleTime=-1
  Display : Display
  Multiport Switch1 : MultiPortSwitch  DataPortOrder=Zero-based contiguous  Inputs=29  DataPortForDefault=Additional data port  DiagnosticForDefault=Warning  zeroidx=on  SaturateOnIntegerOverflow=off  InputSameDT=off
  Scope : Scope
  Subtract : Sum  Inputs=+-  OutDataTypeStr=uint8  AccumDataTypeStr=uint8  RndMeth=Simplest  SaturateOnIntegerOverflow=on
  out : Outport
  wires:
  Multiport Switch1/1 -> out/1
  CTR/1 -> Subtract/2
  Bit Shift27/1 -> Multiport Switch1/30
  Bit Shift26/1 -> Multiport Switch1/29
  Bit Shift25/1 -> Multiport Switch1/28
  Bit Shift24/1 -> Multiport Switch1/27
  Bit Shift23/1 -> Multiport Switch1/26
  Bit Shift22/1 -> Multiport Switch1/25
  Bit Shift21/1 -> Multiport Switch1/24
  Bit Shift20/1 -> Multiport Switch1/23
  Bit Shift19/1 -> Multiport Switch1/22
  Bit Shift18/1 -> Multiport Switch1/21
  Bit Shift17/1 -> Multiport Switch1/20
  Bit Shift16/1 -> Multiport Switch1/19
  Bit Shift15/1 -> Multiport Switch1/18
  Bit Shift14/1 -> Multiport Switch1/17
  Bit Shift13/1 -> Multiport Switch1/16
  Bit Shift12/1 -> Multiport Switch1/15
  Bit Shift11/1 -> Multiport Switch1/14
  Bit Shift10/1 -> Multiport Switch1/13
  Bit Shift9/1 -> Multiport Switch1/12
  Bit Shift8/1 -> Multiport Switch1/11
  Bit Shift7/1 -> Multiport Switch1/10
  Bit Shift6/1 -> Multiport Switch1/9
  Bit Shift5/1 -> Multiport Switch1/8
  Bit Shift4/1 -> Multiport Switch1/7
  Bit Shift3/1 -> Multiport Switch1/6
  in/1 -> Multiport Switch1/31, Multiport Switch1/3, Multiport Switch1/4, Multiport Switch1/5, Bit Shift26/1, Bit Shift27/1, Bit Shift25/1, Bit Shift24/1, Bit Shift23/1, Bit Shift22/1, Bit Shift21/1, Bit Shift20/1, Bit Shift19/1, Bit Shift18/1, Bit Shift17/1, Bit Shift16/1, Bit Shift15/1, Bit Shift14/1, Bit Shift13/1, Bit Shift12/1, Bit Shift11/1, Bit Shift10/1, Bit Shift9/1, Bit Shift8/1, Bit Shift7/1, Bit Shift6/1, Bit Shift5/1, Bit Shift4/1, Bit Shift3/1, Multiport Switch1/2
  in1/1 -> Add/2
  Constant1/1 -> Add/1
  Subtract/1 -> Display/1, Multiport Switch1/1, Scope/1
  Add/1 -> Subtract/1

== system UZ_EnDat_be4_optimizing_agaib/UZ_ENDAT/ManualSerialize/padding2 ==
  in : Inport
  Bit Shift2 : hdlsllib/Logic and Bit Operations/Bit Shift  mode=Shift Right Logical  N=1
  Bit Slice2 : hdlsllib/Logic and Bit Operations/Bit Slice  lidx=0  ridx=0
  Data Type Conversion2 : DataTypeConversion  OutDataTypeStr=boolean  RndMeth=Nearest  SaturateOnIntegerOverflow=off
  Switch2 : Switch  Criteria=u2 > Threshold  SaturateOnIntegerOverflow=off  InputSameDT=off
  out : Outport
  wires:
  in/1 -> Bit Shift2/1, Switch2/1, Bit Slice2/1
  Bit Shift2/1 -> Switch2/3
  Data Type Conversion2/1 -> Switch2/2
  Bit Slice2/1 -> Data Type Conversion2/1
  Switch2/1 -> out/1

== system UZ_EnDat_be4_optimizing_agaib/UZ_ENDAT/ManualSerialize/padding5 ==
  in : Inport
  Bit Shift1 : hdlsllib/Logic and Bit Operations/Bit Shift  mode=Shift Right Logical  N=2
  Bit Shift2 : hdlsllib/Logic and Bit Operations/Bit Shift  mode=Shift Right Logical  N=1
  Bit Shift3 : hdlsllib/Logic and Bit Operations/Bit Shift  mode=Shift Right Logical  N=3
  Bit Slice1 : hdlsllib/Logic and Bit Operations/Bit Slice  lidx=0  ridx=0
  Bit Slice3 : hdlsllib/Logic and Bit Operations/Bit Slice  lidx=1  ridx=0
  Bit Slice4 : hdlsllib/Logic and Bit Operations/Bit Slice  lidx=2  ridx=0
  Compare To Zero : hdlsllib/Logic and Bit Operations/Compare To Zero  relop=<=  OutDataTypeStr=boolean
  Compare To Zero1 : hdlsllib/Logic and Bit Operations/Compare To Zero  relop=<=  OutDataTypeStr=boolean
  Compare To Zero2 : hdlsllib/Logic and Bit Operations/Compare To Zero  relop=<=  OutDataTypeStr=boolean
  Logical Operator : Logic  Inputs=3  AllPortsSameDT=off  OutDataTypeStr=boolean
  Logical Operator1 : Logic  Operator=NOT  Inputs=3  AllPortsSameDT=off  OutDataTypeStr=boolean
  Logical Operator2 : Logic  Operator=NOT  Inputs=3  AllPortsSameDT=off  OutDataTypeStr=boolean
  Logical Operator3 : Logic  Inputs=3  AllPortsSameDT=off  OutDataTypeStr=boolean
  Logical Operator4 : Logic  Inputs=3  AllPortsSameDT=off  OutDataTypeStr=boolean
  Switch1 : Switch  Criteria=u2 > Threshold  SaturateOnIntegerOverflow=off  InputSameDT=off
  Switch2 : Switch  Criteria=u2 > Threshold  SaturateOnIntegerOverflow=off  InputSameDT=off
  Switch3 : Switch  Criteria=u2 > Threshold  SaturateOnIntegerOverflow=off  InputSameDT=off
  out : Outport
  wires:
  in/1 -> Bit Slice4/1, Bit Slice3/1, Bit Slice1/1, Switch2/3, Bit Shift2/1
  Bit Shift2/1 -> Switch2/1
  Switch2/1 -> Switch1/3, Bit Shift1/1
  Bit Slice3/1 -> Compare To Zero/1
  Bit Slice4/1 -> Compare To Zero1/1
  Bit Slice1/1 -> Compare To Zero2/1
  Compare To Zero2/1 -> Logical Operator4/2, Logical Operator3/1, Logical Operator/1
  Compare To Zero/1 -> Logical Operator4/1, Logical Operator3/2, Logical Operator1/1
  Logical Operator1/1 -> Logical Operator/3
  Compare To Zero1/1 -> Logical Operator4/3, Logical Operator2/1
  Logical Operator2/1 -> Logical Operator/2, Logical Operator3/3
  Logical Operator/1 -> Switch2/2
  Bit Shift1/1 -> Switch1/1
  Logical Operator3/1 -> Switch1/2
  Switch1/1 -> Switch3/3, Bit Shift3/1
  Bit Shift3/1 -> Switch3/1
  Logical Operator4/1 -> Switch3/2
  Switch3/1 -> out/1

== system UZ_EnDat_be4_optimizing_agaib/UZ_ENDAT/ManualSerialize/prolonger ==
  in : Inport
  Delay4 : Delay  DelayLength=1
  Logical Operator5 : Logic  Operator=OR  AllPortsSameDT=off  OutDataTypeStr=boolean
  out : Outport
  wires:
  Logical Operator5/1 -> out/1
  in/1 -> Delay4/1, Logical Operator5/1
  Delay4/1 -> Logical Operator5/2

== system UZ_EnDat_be4_optimizing_agaib/UZ_ENDAT/ManualSerialize1/FF1 ==
  SET : Inport
  RST : Inport  Port=2
  S-R Flip-Flop : simulink_extras/Flip Flops/S-R Flip-Flop  initial_condition=0
  OQ : Outport
  NOQ : Outport  Port=2
  wires:
  SET/1 -> S-R Flip-Flop/1
  RST/1 -> S-R Flip-Flop/2
  S-R Flip-Flop/1 -> OQ/1
  S-R Flip-Flop/2 -> NOQ/1

== system UZ_EnDat_be4_optimizing_agaib/UZ_ENDAT/ManualSerialize1/SetZero64modified ==
  valin : Inport
  setzero : Inport  Port=2  OutDataTypeStr=boolean
  Trigger : TriggerPort  TriggerType=either  VariantControl=(inherit)
  Constant2 : Constant  Value=0  OutDataTypeStr=uint64  SampleTime=-1
  Index Vector1 : MultiPortSwitch  DataPortOrder=Zero-based contiguous  Inputs=2  zeroidx=on  OutDataTypeStr=uint64  SaturateOnIntegerOverflow=off  InputSameDT=off
  valueout : Outport  InitialOutput=1  VectorParamsAs1DForOutWhenUnconnected=off
  wires:
  valin/1 -> Index Vector1/2
  Index Vector1/1 -> valueout/1
  Constant2/1 -> Index Vector1/3
  setzero/1 -> Index Vector1/1

== system UZ_EnDat_be4_optimizing_agaib/UZ_ENDAT/ManualSerialize1/Storage1 ==
  Data : Inport
  Write : Inport  Port=2  OutDataTypeStr=boolean
  Compare To Zero : hdlsllib/Logic and Bit Operations/Compare To Zero  relop===  OutDataTypeStr=boolean
  Delay2 : Delay  DelayLength=1
  Logical Operator1 : Logic  AllPortsSameDT=off  OutDataTypeStr=boolean
  Logical Operator2 : Logic  Operator=NOT  AllPortsSameDT=off  OutDataTypeStr=boolean
  Single Port RAM System : hdlsllib/HDL RAMs/Single Port RAM System  Commented=on  RAMType=Single port  AsyncRead=off  WriteOutputValue=Old data  RAMInitialValue=0  allowBusInputs=off  WritesHaveOutput=on  NumReads=0  NumWrites=1  SimulateUsing=Code generation
  Switch : Switch  Criteria=u2 > Threshold  SaturateOnIntegerOverflow=off  InputSameDT=off
  prolonger : Subsystem  Commented=through
  out : Outport
  wrok : Outport  Port=2  OutDataTypeStr=boolean
  wires:
  Switch/1 -> Delay2/1
  Compare To Zero/1 -> Logical Operator2/1
  Logical Operator2/1 -> Logical Operator1/2
  prolonger/1(out) -> wrok/1
  Data/1 -> Compare To Zero/1, Switch/1
  Delay2/1 -> out/1, Switch/3
  Logical Operator1/1 -> prolonger/1(in), Switch/2
  Write/1 -> Logical Operator1/1

== system UZ_EnDat_be4_optimizing_agaib/UZ_ENDAT/ManualSerialize1/Storage16 ==
  Data : Inport
  Write : Inport  Port=2  OutDataTypeStr=boolean
  Compare To Zero : hdlsllib/Logic and Bit Operations/Compare To Zero  relop===  OutDataTypeStr=boolean
  Logical Operator : Logic  Operator=NOT  AllPortsSameDT=off  OutDataTypeStr=boolean
  Logical Operator1 : Logic  Inputs=3  AllPortsSameDT=off  OutDataTypeStr=boolean
  Logical Operator2 : Logic  Operator=NOT  AllPortsSameDT=off  OutDataTypeStr=boolean
  Logical Operator3 : Logic  Inputs=3  AllPortsSameDT=off  OutDataTypeStr=boolean
  Logical Operator4 : Logic  Operator=NOT  AllPortsSameDT=off  OutDataTypeStr=boolean
  Relational Operator : RelationalOperator  Operator===  OutDataTypeStr=boolean  InputSameDT=off
  Scope : Scope  NumInputPorts=5
  Single Port RAM System : hdlsllib/HDL RAMs/Single Port RAM System  RAMType=Single port  AsyncRead=off  WriteOutputValue=Old data  RAMInitialValue=0  allowBusInputs=off  WritesHaveOutput=on  NumReads=0  NumWrites=1  SimulateUsing=Code generation
  adress : Constant  Value=6  OutDataTypeStr=uint8  SampleTime=-1
  out : Outport
  wrok : Outport  Port=2  OutDataTypeStr=boolean
  wires:
  Single Port RAM System/1 -> Relational Operator/1, out/1
  Data/1 -> Compare To Zero/1, Single Port RAM System/1, Relational Operator/2
  adress/1 -> Single Port RAM System/2
  Relational Operator/1 -> Scope/1, Logical Operator/1, Logical Operator3/1
  Logical Operator/1 -> Logical Operator1/2
  Write/1 -> Scope/4, Logical Operator4/1, Logical Operator1/1
  Compare To Zero/1 -> Logical Operator2/1
  Logical Operator1/1 -> Single Port RAM System/3, Scope/5
  Logical Operator3/1 -> wrok/1, Scope/2
  Logical Operator4/1 -> Logical Operator3/3
  Logical Operator2/1 -> Logical Operator1/3, Logical Operator3/2, Scope/3

== system UZ_EnDat_be4_optimizing_agaib/UZ_ENDAT/ManualSerialize1/Storage2 ==
  Data : Inport
  Write : Inport  Port=2  OutDataTypeStr=boolean
  Compare To Zero : hdlsllib/Logic and Bit Operations/Compare To Zero  relop===  OutDataTypeStr=boolean
  Delay : Delay  DelayLength=1
  Delay2 : Delay  DelayLength=1
  Logical Operator1 : Logic  AllPortsSameDT=off  OutDataTypeStr=boolean
  Logical Operator2 : Logic  Operator=NOT  AllPortsSameDT=off  OutDataTypeStr=boolean
  Scope1 : Scope  NumInputPorts=2
  Single Port RAM System : hdlsllib/HDL RAMs/Single Port RAM System  Commented=on  RAMType=Single port  AsyncRead=off  WriteOutputValue=Old data  RAMInitialValue=0  allowBusInputs=off  WritesHaveOutput=on  NumReads=0  NumWrites=1  SimulateUsing=Code generation
  Switch : Switch  Criteria=u2 > Threshold  SaturateOnIntegerOverflow=off  InputSameDT=off
  prolonger : Subsystem
  out : Outport
  wrok : Outport  Port=2  OutDataTypeStr=boolean
  wires:
  Switch/1 -> Delay2/1
  Compare To Zero/1 -> Logical Operator2/1
  Logical Operator1/1 -> Delay/1, Switch/2
  Logical Operator2/1 -> Logical Operator1/2
  prolonger/1(out) -> wrok/1
  Data/1 -> Scope1/1, Compare To Zero/1, Switch/1
  Delay2/1 -> out/1, Switch/3
  Delay/1 -> prolonger/1(in)
  Write/1 -> Logical Operator1/1
